simulink model "task_5"  (R2023a)
settings: Solver=VariableStepAuto  StartTime=0.0  StopTime=10.0  RelTol=1e-8
settings Model: Creator=user  LastModifiedBy=user

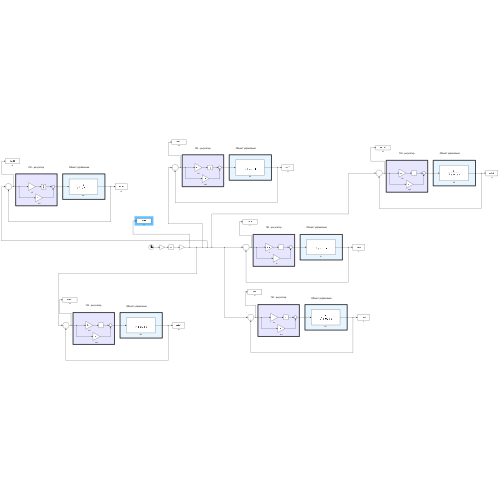
[thumbnail: Simulink's stored preview of the top-level diagram]
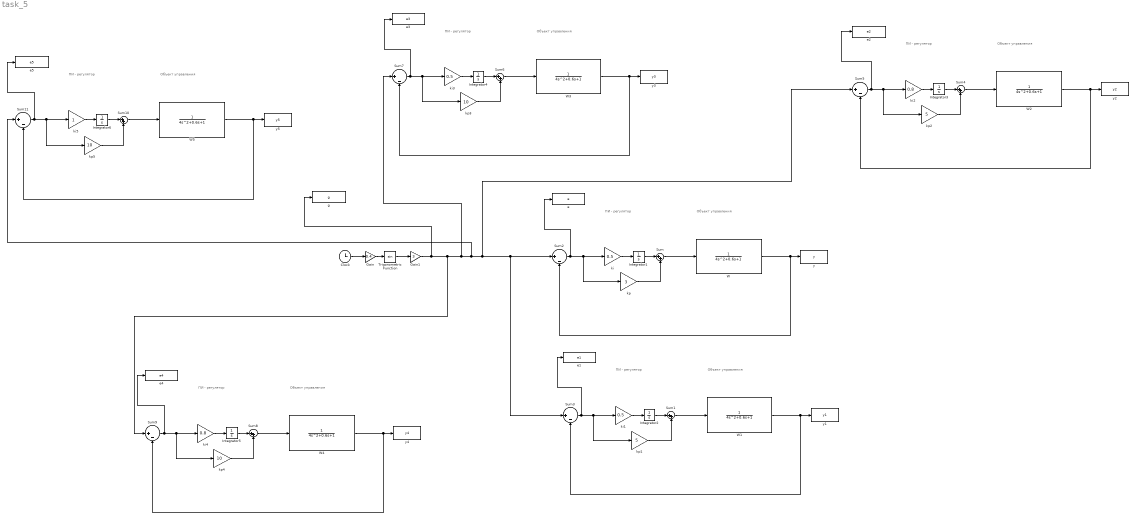
== system task_5 ==
  note: ПИ - регулятор
  note: Объект управления
  note: Объект управления
  note: ПИ - регулятор
  note: Объект управления
  note: ПИ - регулятор
  note: Объект управления
  note: ПИ - регулятор
  note: Объект управления
  note: ПИ - регулятор
  note: Объект управления
  note: ПИ - регулятор
  Clock : Clock
  Gain : Gain  Gain=0.4
  Gain1 : Gain  Gain=3
  Integrator{1..6} (6 alike) : Integrator
  Sum{,1,4,6,8,10} (6 alike) : Sum  Inputs=|++
  Sum{2..3,5,7,9,11} (6 alike) : Sum  Inputs=|+-
  Trigonometric Function : Trigonometry
  W{,1..5} (6 alike) : TransferFcn  Denominator=[4 0.6 1]
  e : ToWorkspace  VariableName=e  SaveFormat=Timeseries  SampleTime=-1
  e1 : ToWorkspace  VariableName=e1  SaveFormat=Timeseries  SampleTime=-1
  e2 : ToWorkspace  VariableName=e2  SaveFormat=Timeseries  SampleTime=-1
  e3 : ToWorkspace  VariableName=e3  SaveFormat=Timeseries  SampleTime=-1
  e4 : ToWorkspace  VariableName=e4  SaveFormat=Timeseries  SampleTime=-1
  e5 : ToWorkspace  VariableName=e5  SaveFormat=Timeseries  SampleTime=-1
  g : ToWorkspace  VariableName=g  SaveFormat=Timeseries  SampleTime=-1
  ki : Gain  Gain=0.5
  ki1 : Gain  Gain=0.5
  ki2 : Gain  Gain=0.8
  ki3 : Gain  Gain=0.5
  ki4 : Gain  Gain=0.8
  ki5 : Gain
  kp : Gain  Gain=3
  kp1 : Gain  Gain=5
  kp2 : Gain  Gain=5
  kp3 : Gain  Gain=10
  kp4 : Gain  Gain=10
  kp5 : Gain  Gain=10
  y : ToWorkspace  VariableName=y  SaveFormat=Timeseries  SampleTime=-1
  y1 : ToWorkspace  VariableName=y1  SaveFormat=Timeseries  SampleTime=-1
  y2 : ToWorkspace  VariableName=y2  SaveFormat=Timeseries  SampleTime=-1
  y3 : ToWorkspace  VariableName=y3  SaveFormat=Timeseries  SampleTime=-1
  y4 : ToWorkspace  VariableName=y4  SaveFormat=Timeseries  SampleTime=-1
  y5 : ToWorkspace  VariableName=y5  SaveFormat=Timeseries  SampleTime=-1
  wires:
  ki/1 -> Integrator1/1
  Sum2/1 -> kp/1, ki/1, e/1
  W/1 -> Sum2/2, y/1
  Integrator1/1 -> Sum/1
  Sum/1 -> W/1
  kp/1 -> Sum/2
  Clock/1 -> Gain/1
  Integrator2/1 -> Sum1/1
  kp1/1 -> Sum1/2
  ki1/1 -> Integrator2/1
  Sum3/1 -> kp1/1, ki1/1, e1/1
  Sum1/1 -> W1/1
  W1/1 -> Sum3/2, y1/1
  Integrator3/1 -> Sum4/1
  kp2/1 -> Sum4/2
  ki2/1 -> Integrator3/1
  Sum5/1 -> kp2/1, ki2/1, e2/1
  Sum4/1 -> W2/1
  W2/1 -> Sum5/2, y2/1
  Integrator4/1 -> Sum6/1
  kp3/1 -> Sum6/2
  ki3/1 -> Integrator4/1
  Sum7/1 -> kp3/1, ki3/1, e3/1
  Sum6/1 -> W3/1
  W3/1 -> Sum7/2, y3/1
  Integrator5/1 -> Sum8/1
  kp4/1 -> Sum8/2
  ki4/1 -> Integrator5/1
  Sum9/1 -> kp4/1, ki4/1, e4/1
  Sum8/1 -> W4/1
  W4/1 -> Sum9/2, y4/1
  Integrator6/1 -> Sum10/1
  kp5/1 -> Sum10/2
  ki5/1 -> Integrator6/1
  Sum11/1 -> kp5/1, ki5/1, e5/1
  Sum10/1 -> W5/1
  Gain/1 -> Trigonometric Function/1
  W5/1 -> Sum11/2, y5/1
  Trigonometric Function/1 -> Gain1/1
  Gain1/1 -> g/1, Sum9/1, Sum7/1, Sum11/1, Sum5/1, Sum3/1, Sum2/1
